simulink model "rotacional_simulink"  (R2024a)
settings: Solver=ode4  StartTime=0.0  StopTime=10  FixedStep=0.001  RelTol=1e-3
values from neighbouring files (symbols this model uses):
  k = 100    [Parametros_rotacional.m]    (also in rota.m)
  m = 10    [Parametros_rotacional.m]    (also in rota.m)
settings Model: Creator=ferch  LastModifiedBy=100117273
settings OptimizationCC: ReuseModelBlockBuffer=off
settings RTWCC: GPUComputeCapability=3.5

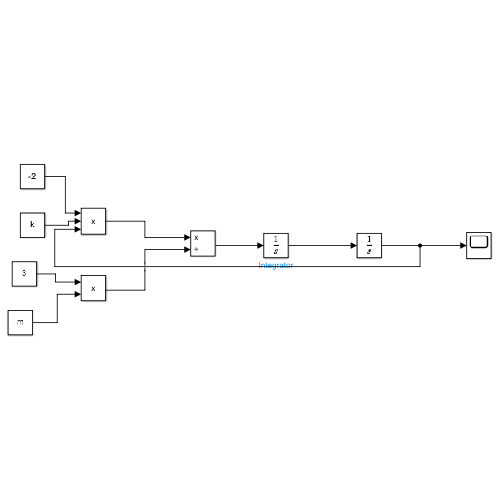
[thumbnail: Simulink's stored preview of the top-level diagram]
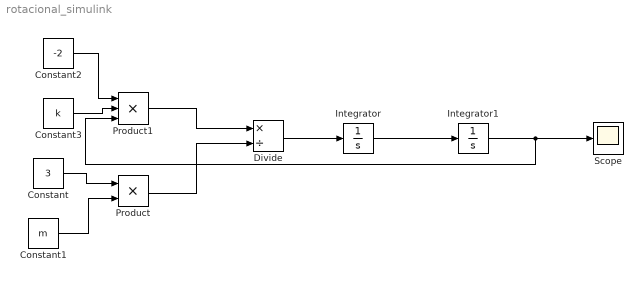
== system rotacional_simulink ==
  Constant : Constant  Value=3
  Constant1 : Constant  Value=m
  Constant2 : Constant  Value=-2
  Constant3 : Constant  Value=k
  Divide : Product  Inputs=*/
  Integrator : Integrator  InitialCondition=2
  Integrator1 : Integrator
  Product : Product
  Product1 : Product  Inputs=3
  Scope : Scope
  wires:
  Integrator/1 -> Integrator1/1
  Integrator1/1 -> Product1/3, Scope/1
  Divide/1 -> Integrator/1
  Product1/1 -> Divide/1
  Product/1 -> Divide/2
  Constant/1 -> Product/1
  Constant1/1 -> Product/2
  Constant2/1 -> Product1/1
  Constant3/1 -> Product1/2
